simulink library "ePTO"  (R2016a)
settings: Solver=ode45  StartTime=0.0  StopTime=10.0  RelTol=1e-3
undefined symbols (not defined in the file): AWR_InvStError, drvEmot_AWR_InvStError, ePTO, ePTO_baseLoad_enable, ePTO_baseLoad_lutData_power, ePTO_baseLoad_lutIdx_tamb, ePTO_coolingBox_coolingPowerOn, ePTO_coolingBox_coolingPowerStandby, ePTO_coolingBox_enable, ePTO_coolingBox_height, ePTO_coolingBox_isRigid, ePTO_coolingBox_length, ePTO_coolingBox_lowerTemp, ePTO_coolingBox_tempInit, ePTO_coolingBox_tires_rdynTrailer, ePTO_coolingBox_upperTemp, ePTO_coolingBox_width, ePTO_posBasedActivatedConsumer_enable, ePTO_posBasedActivatedConsumer_types, ePTO_triggerBasedActivatedConsumer_enable, ePTO_triggerBasedActivatedConsumer_types
libraries: simulink x5
settings Model: Creator=ORNOVNU  LastModifiedBy=HJAGADI
settings DataIOCC: LimitDataPoints=on  SaveFormat=StructureWithTime
settings HardwareCC: ProdWordSize=32  ProdHWDeviceType=Specified

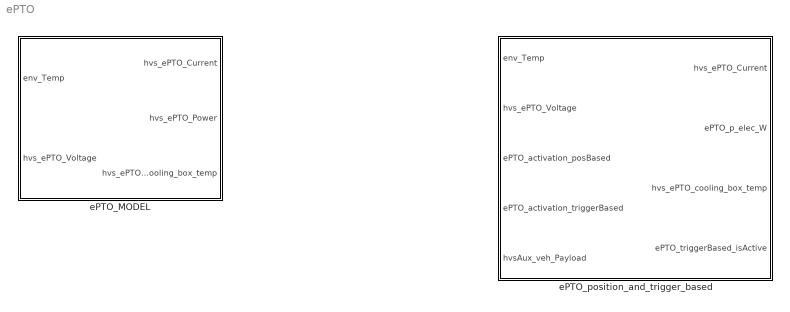
== system ePTO ==
  ePTO_MODEL : Subsystem
  ePTO_position_and_trigger_based : Subsystem

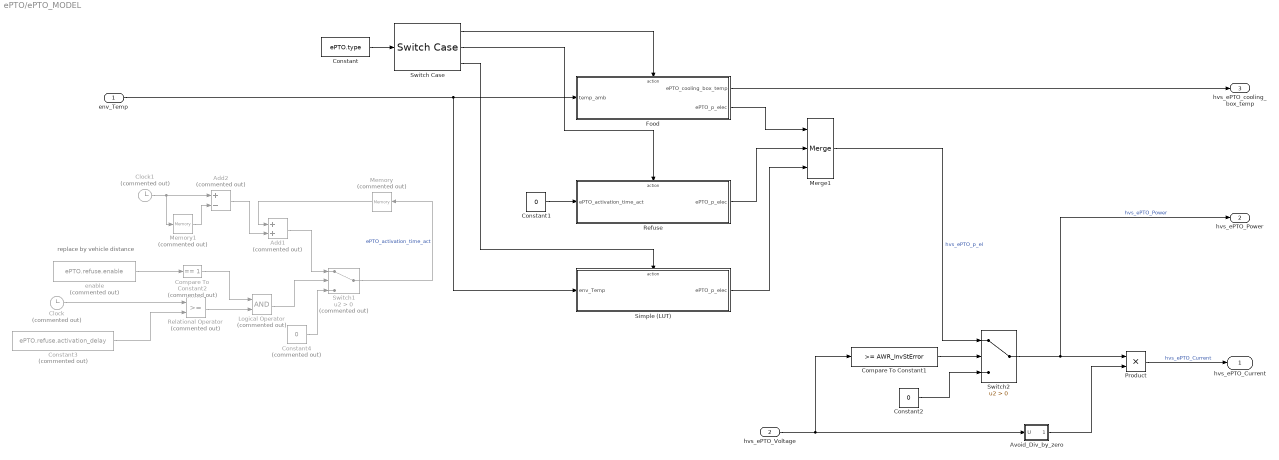
== system ePTO/ePTO_MODEL ==
  note: replace by vehicle distance
  env_Temp : Inport
  hvs_ePTO_Voltage : Inport  Port=2
  Add1 : Sum  Commented=on
  Add2 : Sum  Commented=on  Inputs=+-
  Avoid_Div_by_zero : Subsystem
  Clock : Clock  Commented=on
  Clock1 : Clock  Commented=on
  Compare To Constant1 : simulink/Logic and Bit Operations/Compare To Constant  relop=>=  const=AWR_InvStError  OutDataTypeStr=boolean
  Compare To Constant2 : simulink/Logic and Bit Operations/Compare To Constant  Commented=on  relop===  const=1  OutDataTypeStr=boolean
  Constant : Constant  Value=ePTO.type
  Constant1 : Constant  Value=0
  Constant2 : Constant  Value=0
  Constant3 : Constant  Commented=on  Value=ePTO.refuse.activation_delay
  Constant4 : Constant  Commented=on  Value=0
  Food : Subsystem  TreatAsAtomicUnit=on
  Logical Operator : Logic  Commented=on  AllPortsSameDT=off  OutDataTypeStr=boolean
  Memory : Memory  Commented=on
  Memory1 : Memory  Commented=on
  Merge1 : Merge  Inputs=3
  Product : Product
  Refuse : Subsystem  TreatAsAtomicUnit=on
  Relational Operator : RelationalOperator  Commented=on  OutDataTypeStr=boolean
  Simple (LUT) : Subsystem  TreatAsAtomicUnit=on
  Switch Case : SwitchCase  CaseConditions={1,2}
  Switch1 : Switch  Commented=on  Criteria=u2 > Threshold
  Switch2 : Switch  Criteria=u2 > Threshold
  enable : Constant  Commented=on  Value=ePTO.refuse.enable
  hvs_ePTO_Current : Outport
  hvs_ePTO_Power : Outport  Port=2
  hvs_ePTO_cooling_box_temp : Outport  Port=3
  wires:
  Constant/1 -> Switch Case/1
  Switch Case/1 -> Food/Action
  Switch Case/2 -> Refuse/Action
  Refuse/1(ePTO_p_elec) -> Merge1/2
  Switch1/1 -> Memory/1  "ePTO_activation_time_act"
  enable/1 -> Compare To Constant2/1
  Clock/1 -> Relational Operator/1
  Constant3/1 -> Relational Operator/2
  Constant4/1 -> Switch1/3
  Logical Operator/1 -> Switch1/2
  Relational Operator/1 -> Logical Operator/2
  Compare To Constant2/1 -> Logical Operator/1
  Add2/1 -> Add1/2
  Clock1/1 -> Memory1/1, Add2/1
  Memory1/1 -> Add2/2
  Add1/1 -> Switch1/1
  Memory/1 -> Add1/1
  Constant1/1 -> Refuse/1(ePTO_activation_time_act)
  env_Temp/1 -> Simple (LUT)/1(env_Temp), Food/1(temp_amb)
  Food/2(ePTO_p_elec) -> Merge1/1
  Merge1/1 -> Switch2/1  "hvs_ePTO_p_el"
  Product/1 -> hvs_ePTO_Current/1  "hvs_ePTO_Current"
  Compare To Constant1/1 -> Switch2/2
  Constant2/1 -> Switch2/3
  Food/1(ePTO_cooling_box_temp) -> hvs_ePTO_cooling_box_temp/1
  Switch2/1 -> hvs_ePTO_Power/1, Product/1  "hvs_ePTO_Power"
  hvs_ePTO_Voltage/1 -> Avoid_Div_by_zero/1(U), Compare To Constant1/1
  Avoid_Div_by_zero/1(1/U) -> Product/2
  Switch Case/3 -> Simple (LUT)/Action
  Simple (LUT)/1(ePTO_p_elec) -> Merge1/3

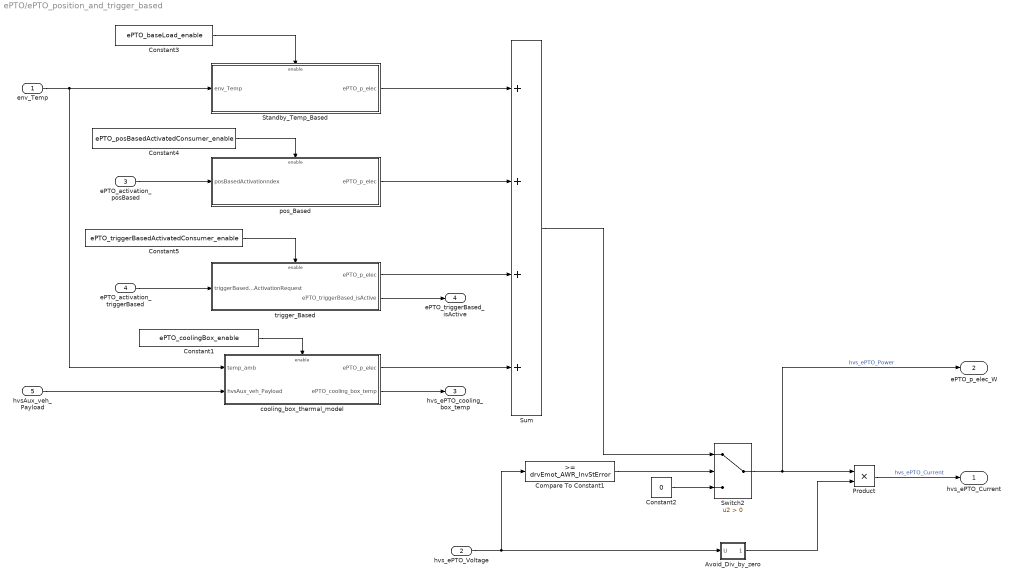
== system ePTO/ePTO_position_and_trigger_based ==
  env_Temp : Inport
  hvs_ePTO_Voltage : Inport  Port=2
  ePTO_activation_posBased : Inport  Port=3
  ePTO_activation_triggerBased : Inport  Port=4
  hvsAux_veh_Payload : Inport  Port=5
  Avoid_Div_by_zero : Subsystem
  Compare To Constant1 : simulink/Logic and Bit Operations/Compare To Constant  relop=>=  const=drvEmot_AWR_InvStError  OutDataTypeStr=boolean
  Constant1 : Constant  Value=ePTO_coolingBox_enable
  Constant2 : Constant  Value=0
  Constant3 : Constant  Value=ePTO_baseLoad_enable
  Constant4 : Constant  Value=ePTO_posBasedActivatedConsumer_enable
  Constant5 : Constant  Value=ePTO_triggerBasedActivatedConsumer_enable
  Product : Product
  Standby_Temp_Based : Subsystem
  Sum : Sum  Inputs=++++
  Switch2 : Switch  Criteria=u2 > Threshold
  cooling_box_thermal_model : Subsystem
  pos_Based : Subsystem
  trigger_Based : Subsystem
  hvs_ePTO_Current : Outport
  ePTO_p_elec_W : Outport  Port=2
  hvs_ePTO_cooling_box_temp : Outport  Port=3
  ePTO_triggerBased_isActive : Outport  Port=4
  wires:
  Avoid_Div_by_zero/1(1/U) -> Product/2
  hvs_ePTO_Voltage/1 -> Avoid_Div_by_zero/1(U), Compare To Constant1/1
  Switch2/1 -> ePTO_p_elec_W/1, Product/1  "hvs_ePTO_Power"
  Constant2/1 -> Switch2/3
  Compare To Constant1/1 -> Switch2/2
  Product/1 -> hvs_ePTO_Current/1  "hvs_ePTO_Current"
  ePTO_activation_posBased/1 -> pos_Based/1(posBasedActivationndex)
  ePTO_activation_triggerBased/1 -> trigger_Based/1(triggerBasedActivationRequest)
  Standby_Temp_Based/1(ePTO_p_elec) -> Sum/1
  trigger_Based/1(ePTO_p_elec) -> Sum/3
  pos_Based/1(ePTO_p_elec) -> Sum/2
  Sum/1 -> Switch2/1
  trigger_Based/2(ePTO_triggerBased_isActive) -> ePTO_triggerBased_isActive/1
  env_Temp/1 -> cooling_box_thermal_model/1(temp_amb), Standby_Temp_Based/1(env_Temp)
  Constant3/1 -> Standby_Temp_Based/Enable
  Constant4/1 -> pos_Based/Enable
  Constant5/1 -> trigger_Based/Enable
  hvsAux_veh_Payload/1 -> cooling_box_thermal_model/2(hvsAux_veh_Payload)
  cooling_box_thermal_model/1(ePTO_p_elec) -> Sum/4
  cooling_box_thermal_model/2(ePTO_cooling_box_temp) -> hvs_ePTO_cooling_box_temp/1
  Constant1/1 -> cooling_box_thermal_model/Enable

== system ePTO/ePTO_MODEL/Avoid_Div_by_zero ==
  U : Inport
  Constant : Constant  Value=10^-6
  Divide : Product  Inputs=/*
  Math Function : Math  Operator=square  SaturateOnIntegerOverflow=on
  Sum : Sum  Inputs=++|
  1/U : Outport
  wires:
  Divide/1 -> 1/U/1
  Math Function/1 -> Divide/1
  Sum/1 -> Divide/2, Math Function/1
  Constant/1 -> Sum/1
  U/1 -> Sum/2

== system ePTO/ePTO_MODEL/Food ==
  temp_amb : Inport
  Action Port : ActionPort  ActionType=case
  ePTO.cooling_box.power_init : Memory
  ePTO.cooling_box.temp_init : Memory  X0=ePTO.cooling_box.temp_init
  ePTO_FOOD_POWER_CALC : Subsystem
  resolve_merge_issue : Gain
  ePTO_cooling_box_temp : Outport
  ePTO_p_elec : Outport  Port=2
  wires:
  ePTO_FOOD_POWER_CALC/1(cooling_box_temp_act) -> ePTO.cooling_box.temp_init/1, ePTO_cooling_box_temp/1
  ePTO.cooling_box.temp_init/1 -> ePTO_FOOD_POWER_CALC/2(cooling_box_temp_act_old)
  ePTO_FOOD_POWER_CALC/2(cooling_box_cooling_power_act) -> resolve_merge_issue/1, ePTO.cooling_box.power_init/1
  ePTO.cooling_box.power_init/1 -> ePTO_FOOD_POWER_CALC/3(cooling_box_cooling_power_act_old)
  temp_amb/1 -> ePTO_FOOD_POWER_CALC/1(env_temp)
  resolve_merge_issue/1 -> ePTO_p_elec/1

== system ePTO/ePTO_MODEL/Refuse ==
  ePTO_activation_time_act : Inport
  Action Port : ActionPort  ActionType=case
  ePTO_rotopress_electric_power : Lookup_n-D  NumberOfTableDimensions=1  BreakpointsForDimension1=ePTO.garbage.time  Table=ePTO.garbage.electric_power  ExtrapMethod=Clip  UseLastTableValue=on  RndMeth=Simplest  InputSameDT=on
  ePTO_p_elec : Outport
  wires:
  ePTO_activation_time_act/1 -> ePTO_rotopress_electric_power/1
  ePTO_rotopress_electric_power/1 -> ePTO_p_elec/1

== system ePTO/ePTO_MODEL/Simple (LUT) ==
  env_Temp : Inport
  Action Port : ActionPort  ActionType=default
  1-D Lookup Table : Lookup_n-D  NumberOfTableDimensions=1  BreakpointsForDimension1=ePTO.simple.lutIdx_tamb  Table=ePTO.simple.lutData_power  ExtrapMethod=Clip  InternalRulePriority=Speed  RndMeth=Simplest  InputSameDT=on
  ePTO_p_elec : Outport
  wires:
  1-D Lookup Table/1 -> ePTO_p_elec/1
  env_Temp/1 -> 1-D Lookup Table/1

== system ePTO/ePTO_position_and_trigger_based/Avoid_Div_by_zero ==
  U : Inport
  Constant : Constant  Value=10^-6
  Divide : Product  Inputs=/*
  Math Function : Math  Operator=square  SaturateOnIntegerOverflow=on
  Sum : Sum  Inputs=++|
  1/U : Outport
  wires:
  U/1 -> Sum/2
  Constant/1 -> Sum/1
  Sum/1 -> Math Function/1, Divide/2
  Math Function/1 -> Divide/1
  Divide/1 -> 1/U/1

== system ePTO/ePTO_position_and_trigger_based/Standby_Temp_Based ==
  env_Temp : Inport
  Enable : EnablePort
  1-D Lookup Table : Lookup_n-D  NumberOfTableDimensions=1  BreakpointsForDimension1=ePTO_baseLoad_lutIdx_tamb  Table=ePTO_baseLoad_lutData_power  ExtrapMethod=Clip  InternalRulePriority=Speed  RndMeth=Simplest  InputSameDT=on
  ePTO_p_elec : Outport
  wires:
  env_Temp/1 -> 1-D Lookup Table/1
  1-D Lookup Table/1 -> ePTO_p_elec/1

== system ePTO/ePTO_position_and_trigger_based/cooling_box_thermal_model ==
  temp_amb : Inport
  hvsAux_veh_Payload : Inport  Port=2
  Enable : EnablePort
  ePTO_FOOD_POWER_CALC : Subsystem
  ePTO_coolingBox_powerInit : Memory  InheritSampleTime=on
  ePTO_coolingBox_tempInit : Memory  X0=ePTO_coolingBox_tempInit  InheritSampleTime=on
  resolve_merge_issue : Gain
  ePTO_p_elec : Outport
  ePTO_cooling_box_temp : Outport  Port=2
  wires:
  ePTO_FOOD_POWER_CALC/1(cooling_box_temp_act) -> ePTO_cooling_box_temp/1, ePTO_coolingBox_tempInit/1
  hvsAux_veh_Payload/1 -> ePTO_FOOD_POWER_CALC/4(hvsAux_veh_Payload)
  resolve_merge_issue/1 -> ePTO_p_elec/1
  ePTO_coolingBox_tempInit/1 -> ePTO_FOOD_POWER_CALC/2(cooling_box_temp_act_old)
  ePTO_FOOD_POWER_CALC/2(cooling_box_cooling_power_act) -> resolve_merge_issue/1, ePTO_coolingBox_powerInit/1
  ePTO_coolingBox_powerInit/1 -> ePTO_FOOD_POWER_CALC/3(cooling_box_cooling_power_act_old)
  temp_amb/1 -> ePTO_FOOD_POWER_CALC/1(env_temp)

== system ePTO/ePTO_position_and_trigger_based/pos_Based ==
  posBasedActivationndex : Inport
  Enable : EnablePort
  Bias : Bias  Bias=-1
  Constant : Constant  Value=0
  Direct Lookup Table (n-D) : LookupNDDirect  NumberOfTableDimensions=1  Table=ePTO_posBasedActivatedConsumer_types
  Saturation1 : Saturate  UpperLimit=99  LowerLimit=1
  Switch : Switch  Criteria=u2 > Threshold
  ePTO_p_elec : Outport
  wires:
  posBasedActivationndex/1 -> Switch/2, Saturation1/1
  Constant/1 -> Switch/3
  Direct Lookup Table (n-D)/1 -> Switch/1
  Switch/1 -> ePTO_p_elec/1
  Bias/1 -> Direct Lookup Table (n-D)/1
  Saturation1/1 -> Bias/1

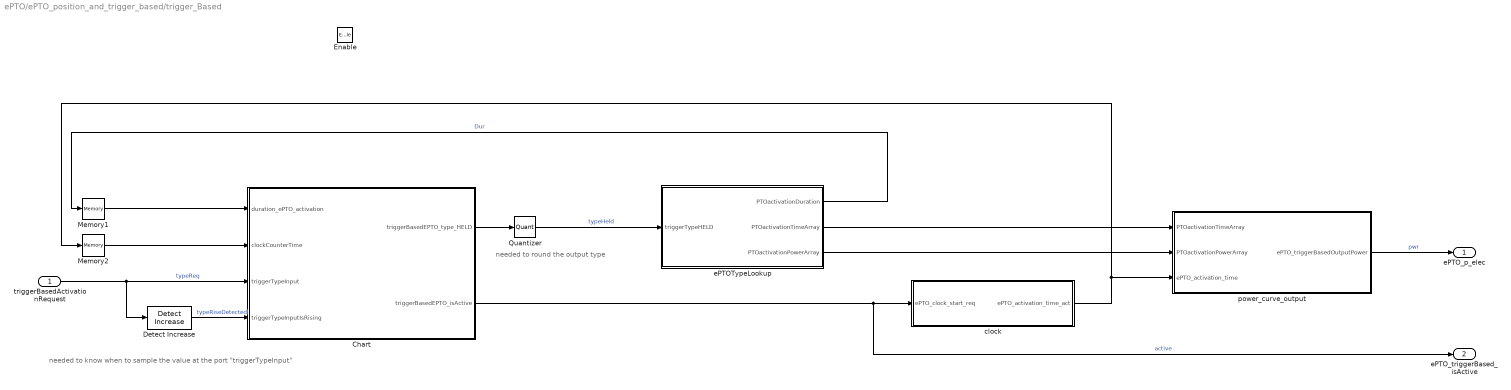
== system ePTO/ePTO_position_and_trigger_based/trigger_Based ==
  note: needed to round the output type
  note: needed to know when to sample the value at the port "triggerTypeInput"
  triggerBasedActivationRequest : Inport
  Enable : EnablePort
  Chart : Stateflow chart  TreatAsAtomicUnit=on
  Detect Increase : simulink/Logic and Bit Operations/Detect Increase  vinit=0.0  OutDataTypeStr=boolean
  Memory1 : Memory  InheritSampleTime=on
  Memory2 : Memory  InheritSampleTime=on
  Quantizer : Quantizer  QuantizationInterval=1
  clock : Subsystem
  ePTOTypeLookup : Subsystem
  power_curve_output : Subsystem
  ePTO_p_elec : Outport
  ePTO_triggerBased_isActive : Outport  Port=2
  wires:
  Memory2/1 -> Chart/2(clockCounterTime)
  clock/1(ePTO_activation_time_act) -> Memory2/1, power_curve_output/3(ePTO_activation_time)
  power_curve_output/1(ePTO_triggerBasedOutputPower) -> ePTO_p_elec/1  "pwr"
  triggerBasedActivationRequest/1 -> Detect Increase/1, Chart/3(triggerTypeInput)  "typeReq"
  ePTOTypeLookup/1(PTOactivationDuration) -> Memory1/1  "Dur"
  ePTOTypeLookup/2(PTOactivationTimeArray) -> power_curve_output/1(PTOactivationTimeArray)
  ePTOTypeLookup/3(PTOactivationPowerArray) -> power_curve_output/2(PTOactivationPowerArray)
  Chart/2(triggerBasedEPTO_isActive) -> ePTO_triggerBased_isActive/1, clock/1(ePTO_clock_start_req)  "active"
  Memory1/1 -> Chart/1(duration_ePTO_activation)
  Chart/1(triggerBasedEPTO_type_HELD) -> Quantizer/1
  Detect Increase/1 -> Chart/4(triggerTypeInputIsRising)  "typeRiseDetected"
  Quantizer/1 -> ePTOTypeLookup/1(triggerTypeHELD)  "typeHeld"

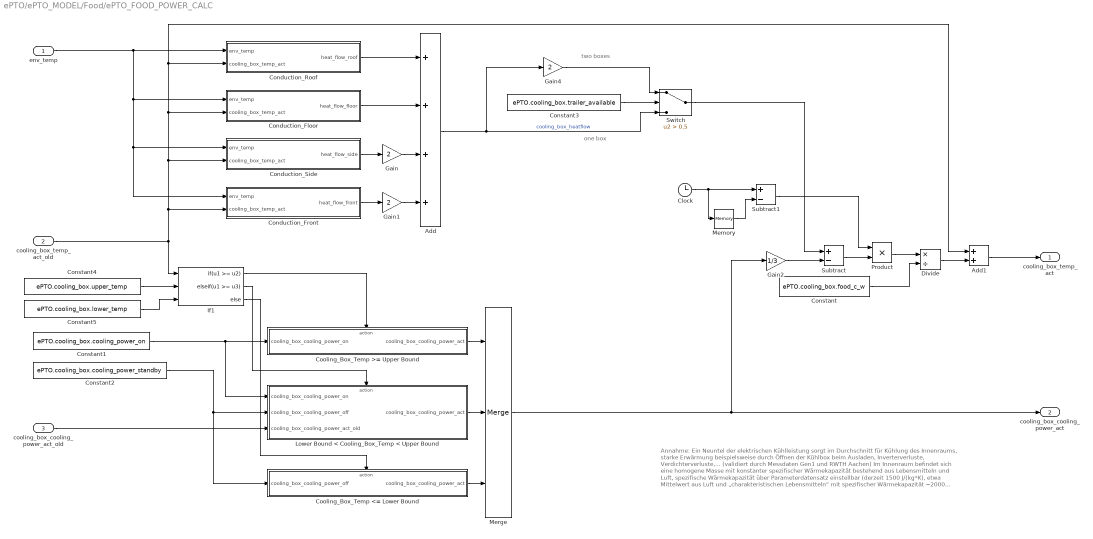
== system ePTO/ePTO_MODEL/Food/ePTO_FOOD_POWER_CALC ==
  note: Annahme: Ein Neuntel der elektrischen Kühlleistung sorgt im Durchschnitt für Kühlung des Innenraums,
      | starke Erwärmung beispielsweise durch Öffnen der Kühlbox beim Ausladen, Inverterverluste, Verdichterverluste,…
      | (validiert durch Messdaten Gen1 und RWTH Aachen)
      |
      | Im Innenraum befindet sich eine homogene Masse mit konstanter spezifischer Wärmekapazität bestehend aus Lebensmitteln und Luft,
      | spezifische Wärmekapazität über Parameterdatensatz einstellbar (derzeit 1500 J/(kg*K),
      | etwa Mittelwert aus Luft und „charakteristischen Lebensmitteln“ mit spezifischer Wärmekapazität ~2000 J/(kg*K)
      |
      | Ref: F. Schuh (TP/EVX)
  note: two boxes
  note: one box
  env_temp : Inport
  cooling_box_temp_act_old : Inport  Port=2
  cooling_box_cooling_power_act_old : Inport  Port=3
  Add : Sum  Inputs=++++
  Add1 : Sum
  Clock : Clock
  Conduction_Floor : Subsystem
  Conduction_Front : Subsystem
  Conduction_Roof : Subsystem
  Conduction_Side : Subsystem
  Constant : Constant  Value=ePTO.cooling_box.food_c_w
  Constant1 : Constant  Value=ePTO.cooling_box.cooling_power_on
  Constant2 : Constant  Value=ePTO.cooling_box.cooling_power_standby
  Constant3 : Constant  Value=ePTO.cooling_box.trailer_available
  Constant4 : Constant  Value=ePTO.cooling_box.upper_temp
  Constant5 : Constant  Value=ePTO.cooling_box.lower_temp
  Cooling_Box_Temp <= Lower Bound : Subsystem  TreatAsAtomicUnit=on
  Cooling_Box_Temp >= Upper Bound : Subsystem  TreatAsAtomicUnit=on
  Divide : Product  Inputs=*/
  Gain : Gain  Gain=2
  Gain1 : Gain  Gain=2
  Gain2 : Gain  Gain=1/3
  Gain4 : Gain  Gain=2
  If1 : If  NumInputs=3  IfExpression=u1 >= u2  ElseIfExpressions=u1 >= u3
  Lower Bound < Cooling_Box_Temp < Upper Bound : Subsystem  TreatAsAtomicUnit=on
  Memory : Memory
  Merge : Merge  Inputs=3
  Product : Product
  Subtract : Sum  Inputs=+-
  Subtract1 : Sum  Inputs=+-
  Switch : Switch  Criteria=u2 > Threshold  Threshold=0.5
  cooling_box_temp_act : Outport
  cooling_box_cooling_power_act : Outport  Port=2
  wires:
  cooling_box_temp_act_old/1 -> If1/1, Conduction_Front/2(cooling_box_temp_act), Conduction_Side/2(cooling_box_temp_act), Conduction_Floor/2(cooling_box_temp_act), Add1/1, Conduction_Roof/2(cooling_box_temp_act)
  Conduction_Side/1(heat_flow_side) -> Gain/1
  Conduction_Front/1(heat_flow_front) -> Gain1/1
  Conduction_Roof/1(heat_flow_roof) -> Add/1
  Conduction_Floor/1(heat_flow_floor) -> Add/2
  Gain/1 -> Add/3
  Gain1/1 -> Add/4
  Add/1 -> Gain4/1, Switch/3  "cooling_box_heatflow"
  Subtract/1 -> Product/2
  Product/1 -> Divide/1
  Constant/1 -> Divide/2
  Divide/1 -> Add1/2
  Add1/1 -> cooling_box_temp_act/1
  If1/1 -> Cooling_Box_Temp >= Upper Bound/Action
  Constant1/1 -> Lower Bound < Cooling_Box_Temp < Upper Bound/1(cooling_box_cooling_power_on), Cooling_Box_Temp >= Upper Bound/1(cooling_box_cooling_power_on)
  If1/2 -> Lower Bound < Cooling_Box_Temp < Upper Bound/Action
  Constant2/1 -> Lower Bound < Cooling_Box_Temp < Upper Bound/2(cooling_box_cooling_power_off), Cooling_Box_Temp <= Lower Bound/1(cooling_box_cooling_power_off)
  If1/3 -> Cooling_Box_Temp <= Lower Bound/Action
  Lower Bound < Cooling_Box_Temp < Upper Bound/1(cooling_box_cooling_power_act) -> Merge/2
  Cooling_Box_Temp >= Upper Bound/1(cooling_box_cooling_power_act) -> Merge/1
  Cooling_Box_Temp <= Lower Bound/1(cooling_box_cooling_power_act) -> Merge/3
  Merge/1 -> cooling_box_cooling_power_act/1, Gain2/1
  Constant3/1 -> Switch/2
  Gain2/1 -> Subtract/2
  env_temp/1 -> Conduction_Floor/1(env_temp), Conduction_Front/1(env_temp), Conduction_Side/1(env_temp), Conduction_Roof/1(env_temp)
  Gain4/1 -> Switch/1
  Switch/1 -> Subtract/1
  Clock/1 -> Memory/1, Subtract1/1
  Memory/1 -> Subtract1/2
  Subtract1/1 -> Product/1
  Constant5/1 -> If1/3
  Constant4/1 -> If1/2
  cooling_box_cooling_power_act_old/1 -> Lower Bound < Cooling_Box_Temp < Upper Bound/3(cooling_box_cooling_power_act_old)

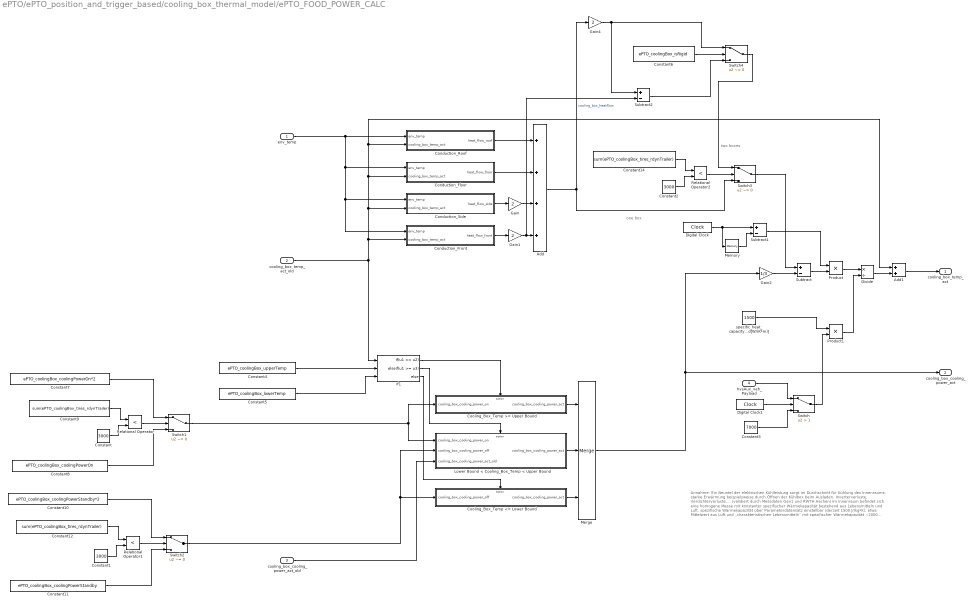
== system ePTO/ePTO_position_and_trigger_based/cooling_box_thermal_model/ePTO_FOOD_POWER_CALC ==
  note: Annahme: Ein Neuntel der elektrischen Kühlleistung sorgt im Durchschnitt für Kühlung des Innenraums,
      | starke Erwärmung beispielsweise durch Öffnen der Kühlbox beim Ausladen, Inverterverluste, Verdichterverluste,…
      | (validiert durch Messdaten Gen1 und RWTH Aachen)
      |
      | Im Innenraum befindet sich eine homogene Masse mit konstanter spezifischer Wärmekapazität bestehend aus Lebensmitteln und Luft,
      | spezifische Wärmekapazität über Parameterdatensatz einstellbar (derzeit 1500 J/(kg*K),
      | etwa Mittelwert aus Luft und „charakteristischen Lebensmitteln“ mit spezifischer Wärmekapazität ~2000 J/(kg*K)
      |
      | Ref: F. Schuh (TP/EVX)
  note: two boxes
  note: one box
  env_temp : Inport
  cooling_box_temp_act_old : Inport  Port=2
  cooling_box_cooling_power_act_old : Inport  Port=3
  hvsAux_veh_Payload : Inport  Port=4
  Add : Sum  Inputs=++++
  Add1 : Sum
  Conduction_Floor : Subsystem
  Conduction_Front : Subsystem
  Conduction_Roof : Subsystem
  Conduction_Side : Subsystem
  Constant : Constant  Value=3000
  Constant1 : Constant  Value=3000
  Constant10 : Constant  Value=ePTO_coolingBox_coolingPowerStandby*2
  Constant11 : Constant  Value=ePTO_coolingBox_coolingPowerStandby
  Constant12 : Constant  Value=sum(ePTO_coolingBox_tires_rdynTrailer)
  Constant14 : Constant  Value=sum(ePTO_coolingBox_tires_rdynTrailer)
  Constant2 : Constant  Value=3000
  Constant3 : Constant  Value=7000
  Constant4 : Constant  Value=ePTO_coolingBox_upperTemp
  Constant5 : Constant  Value=ePTO_coolingBox_lowerTemp
  Constant6 : Constant  Value=ePTO_coolingBox_isRigid
  Constant7 : Constant  Value=ePTO_coolingBox_coolingPowerOn*2
  Constant8 : Constant  Value=ePTO_coolingBox_coolingPowerOn
  Constant9 : Constant  Value=sum(ePTO_coolingBox_tires_rdynTrailer)
  Cooling_Box_Temp <= Lower Bound : Subsystem  TreatAsAtomicUnit=on
  Cooling_Box_Temp >= Upper Bound : Subsystem  TreatAsAtomicUnit=on
  Digital Clock : DigitalClock  SampleTime=-1
  Digital Clock1 : DigitalClock  SampleTime=-1
  Divide : Product  Inputs=*/
  Gain : Gain  Gain=2
  Gain1 : Gain  Gain=2
  Gain2 : Gain  Gain=1/3
  Gain4 : Gain  Gain=2
  If1 : If  NumInputs=3  IfExpression=u1 >= u2  ElseIfExpressions=u1 >= u3
  Lower Bound < Cooling_Box_Temp < Upper Bound : Subsystem  TreatAsAtomicUnit=on
  Memory : Memory  InheritSampleTime=on
  Merge : Merge  Inputs=3
  Product : Product
  Product1 : Product
  Relational Operator : RelationalOperator  Operator=<  OutDataTypeStr=boolean
  Relational Operator1 : RelationalOperator  Operator=<  OutDataTypeStr=boolean
  Relational Operator2 : RelationalOperator  Operator=<  OutDataTypeStr=boolean
  Subtract : Sum  Inputs=+-
  Subtract1 : Sum  Inputs=+-
  Subtract2 : Sum  Inputs=+-
  Switch : Switch  Criteria=u2 > Threshold  Threshold=1
  Switch{1..4} (4 alike) : Switch  Criteria=u2 ~= 0
  specific_heat_capacity_food[W/(K*m)] : Constant  Value=1500
  cooling_box_temp_act : Outport
  cooling_box_cooling_power_act : Outport  Port=2
  wires:
  cooling_box_temp_act_old/1 -> If1/1, Conduction_Front/2(cooling_box_temp_act), Conduction_Side/2(cooling_box_temp_act), Conduction_Floor/2(cooling_box_temp_act), Add1/1, Conduction_Roof/2(cooling_box_temp_act)
  Conduction_Side/1(heat_flow_side) -> Gain/1
  Conduction_Front/1(heat_flow_front) -> Gain1/1
  Conduction_Roof/1(heat_flow_roof) -> Add/1
  Conduction_Floor/1(heat_flow_floor) -> Add/2
  Gain/1 -> Add/3
  Gain1/1 -> Subtract2/2, Add/4
  Add/1 -> Switch3/3, Gain4/1  "cooling_box_heatflow"
  Subtract/1 -> Product/2
  Product/1 -> Divide/1
  Product1/1 -> Divide/2
  Divide/1 -> Add1/2
  Add1/1 -> cooling_box_temp_act/1
  If1/1 -> Cooling_Box_Temp >= Upper Bound/Action
  Switch1/1 -> Lower Bound < Cooling_Box_Temp < Upper Bound/1(cooling_box_cooling_power_on), Cooling_Box_Temp >= Upper Bound/1(cooling_box_cooling_power_on)
  If1/2 -> Lower Bound < Cooling_Box_Temp < Upper Bound/Action
  Switch2/1 -> Lower Bound < Cooling_Box_Temp < Upper Bound/2(cooling_box_cooling_power_off), Cooling_Box_Temp <= Lower Bound/1(cooling_box_cooling_power_off)
  If1/3 -> Cooling_Box_Temp <= Lower Bound/Action
  Lower Bound < Cooling_Box_Temp < Upper Bound/1(cooling_box_cooling_power_act) -> Merge/2
  Cooling_Box_Temp >= Upper Bound/1(cooling_box_cooling_power_act) -> Merge/1
  Cooling_Box_Temp <= Lower Bound/1(cooling_box_cooling_power_act) -> Merge/3
  Merge/1 -> cooling_box_cooling_power_act/1, Gain2/1
  Gain2/1 -> Subtract/2
  env_temp/1 -> Conduction_Floor/1(env_temp), Conduction_Front/1(env_temp), Conduction_Side/1(env_temp), Conduction_Roof/1(env_temp)
  Switch3/1 -> Subtract/1
  Digital Clock/1 -> Memory/1, Subtract1/1
  Memory/1 -> Subtract1/2
  Subtract1/1 -> Product/1
  Constant5/1 -> If1/3
  Constant4/1 -> If1/2
  cooling_box_cooling_power_act_old/1 -> Lower Bound < Cooling_Box_Temp < Upper Bound/3(cooling_box_cooling_power_act_old)
  specific_heat_capacity_food[W/(K*m)]/1 -> Product1/1
  Relational Operator/1 -> Switch1/2
  Constant/1 -> Relational Operator/2
  Constant7/1 -> Switch1/1
  Constant8/1 -> Switch1/3
  Constant9/1 -> Relational Operator/1
  Relational Operator1/1 -> Switch2/2
  Constant1/1 -> Relational Operator1/2
  Constant10/1 -> Switch2/1
  Constant11/1 -> Switch2/3
  Constant12/1 -> Relational Operator1/1
  Relational Operator2/1 -> Switch3/2
  Constant2/1 -> Relational Operator2/2
  Constant14/1 -> Relational Operator2/1
  Digital Clock1/1 -> Switch/2
  hvsAux_veh_Payload/1 -> Switch/1
  Constant3/1 -> Switch/3
  Switch/1 -> Product1/2
  Gain4/1 -> Subtract2/1, Switch4/1
  Switch4/1 -> Switch3/1
  Constant6/1 -> Switch4/2
  Subtract2/1 -> Switch4/3

== system ePTO/ePTO_position_and_trigger_based/trigger_Based/clock ==
  ePTO_clock_start_req : Inport
  Add1 : Sum
  Add2 : Sum  Inputs=+-
  Constant4 : Constant  Value=0
  Digital Clock : DigitalClock  SampleTime=-1
  Memory : Memory  InheritSampleTime=on
  Memory1 : Memory  InheritSampleTime=on
  Switch1 : Switch  Criteria=u2 > Threshold
  ePTO_activation_time_act : Outport
  wires:
  Add1/1 -> Switch1/1
  Memory1/1 -> Add2/2
  Memory/1 -> Add1/1
  Constant4/1 -> Switch1/3
  Switch1/1 -> ePTO_activation_time_act/1, Memory/1  "ePTO_activation_time_act"
  Add2/1 -> Add1/2
  ePTO_clock_start_req/1 -> Switch1/2
  Digital Clock/1 -> Memory1/1, Add2/1

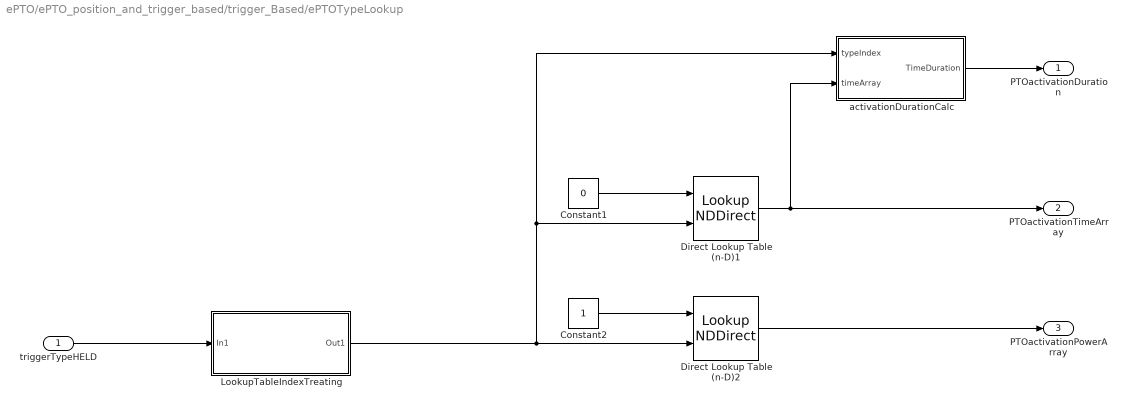
== system ePTO/ePTO_position_and_trigger_based/trigger_Based/ePTOTypeLookup ==
  triggerTypeHELD : Inport
  Constant1 : Constant  Value=0
  Constant2 : Constant
  Direct Lookup Table (n-D)1 : LookupNDDirect  NumberOfTableDimensions=3  InputsSelectThisObjectFromTable=Column  Table=ePTO_triggerBasedActivatedConsumer_types
  Direct Lookup Table (n-D)2 : LookupNDDirect  NumberOfTableDimensions=3  InputsSelectThisObjectFromTable=Column  Table=ePTO_triggerBasedActivatedConsumer_types
  LookupTableIndexTreating : Subsystem
  activationDurationCalc : Subsystem
  PTOactivationDuration : Outport
  PTOactivationTimeArray : Outport  Port=2
  PTOactivationPowerArray : Outport  Port=3
  wires:
  Constant1/1 -> Direct Lookup Table (n-D)1/1
  Constant2/1 -> Direct Lookup Table (n-D)2/1
  Direct Lookup Table (n-D)1/1 -> activationDurationCalc/2(timeArray), PTOactivationTimeArray/1
  Direct Lookup Table (n-D)2/1 -> PTOactivationPowerArray/1
  LookupTableIndexTreating/1(Out1) -> activationDurationCalc/1(typeIndex), Direct Lookup Table (n-D)1/2, Direct Lookup Table (n-D)2/2
  triggerTypeHELD/1 -> LookupTableIndexTreating/1(In1)
  activationDurationCalc/1(TimeDuration) -> PTOactivationDuration/1

== system ePTO/ePTO_position_and_trigger_based/trigger_Based/power_curve_output ==
  PTOactivationTimeArray : Inport
  PTOactivationPowerArray : Inport  Port=2
  ePTO_activation_time : Inport  Port=3
  Lookup Table Dynamic : simulink/Lookup Tables/Lookup Table Dynamic  LookUpMeth=Interpolation-Use End Values  OutDataTypeStr=fixdt('double')  OutputDataTypeScalingMode=Specify via dialog  OutDataType=fixdt('double')  OutScaling=2^-10  DoSatur=off
  ePTO_triggerBasedOutputPower : Outport
  wires:
  ePTO_activation_time/1 -> Lookup Table Dynamic/1
  Lookup Table Dynamic/1 -> ePTO_triggerBasedOutputPower/1
  PTOactivationTimeArray/1 -> Lookup Table Dynamic/2
  PTOactivationPowerArray/1 -> Lookup Table Dynamic/3

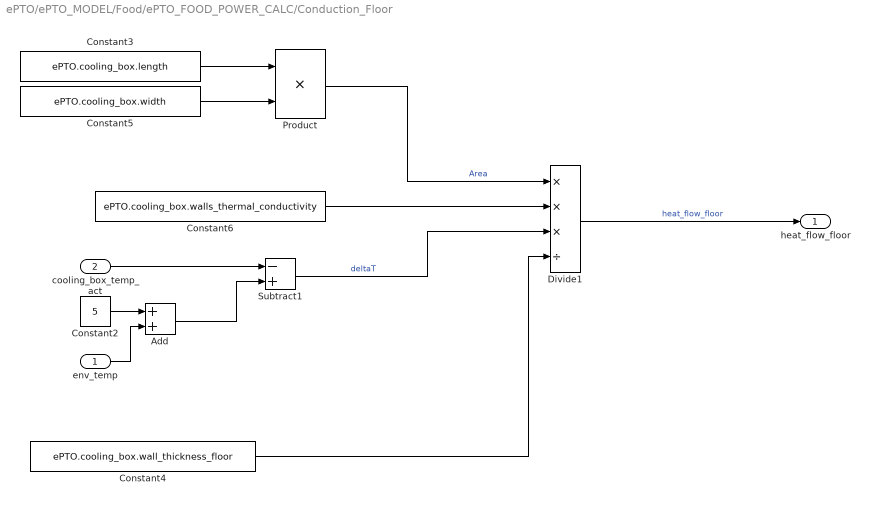
== system ePTO/ePTO_MODEL/Food/ePTO_FOOD_POWER_CALC/Conduction_Floor ==
  env_temp : Inport
  cooling_box_temp_act : Inport  Port=2
  Add : Sum
  Constant2 : Constant  Value=5
  Constant3 : Constant  Value=ePTO.cooling_box.length
  Constant4 : Constant  Value=ePTO.cooling_box.wall_thickness_floor
  Constant5 : Constant  Value=ePTO.cooling_box.width
  Constant6 : Constant  Value=ePTO.cooling_box.walls_thermal_conductivity
  Divide1 : Product  Inputs=***/
  Product : Product
  Subtract1 : Sum  Inputs=-+
  heat_flow_floor : Outport
  wires:
  Divide1/1 -> heat_flow_floor/1  "heat_flow_floor"
  env_temp/1 -> Add/2
  Constant2/1 -> Add/1
  Subtract1/1 -> Divide1/3  "deltaT"
  cooling_box_temp_act/1 -> Subtract1/1
  Product/1 -> Divide1/1  "Area"
  Constant5/1 -> Product/2
  Constant4/1 -> Divide1/4
  Constant3/1 -> Product/1
  Constant6/1 -> Divide1/2
  Add/1 -> Subtract1/2

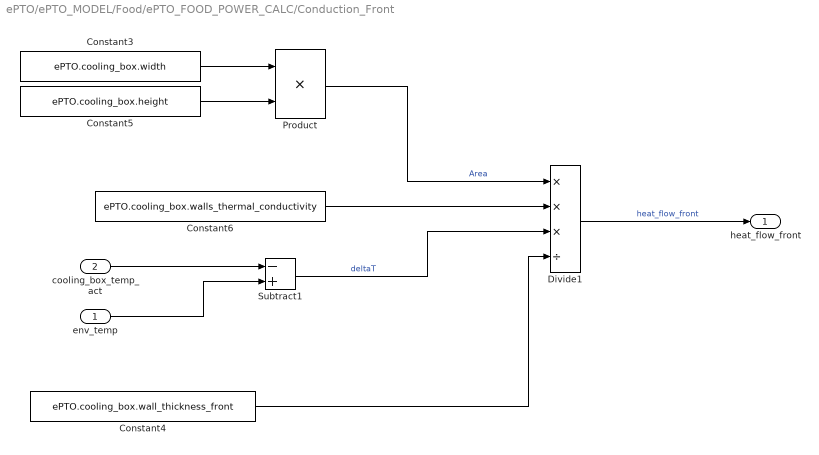
== system ePTO/ePTO_MODEL/Food/ePTO_FOOD_POWER_CALC/Conduction_Front ==
  env_temp : Inport
  cooling_box_temp_act : Inport  Port=2
  Constant3 : Constant  Value=ePTO.cooling_box.width
  Constant4 : Constant  Value=ePTO.cooling_box.wall_thickness_front
  Constant5 : Constant  Value=ePTO.cooling_box.height
  Constant6 : Constant  Value=ePTO.cooling_box.walls_thermal_conductivity
  Divide1 : Product  Inputs=***/
  Product : Product
  Subtract1 : Sum  Inputs=-+
  heat_flow_front : Outport
  wires:
  env_temp/1 -> Subtract1/2
  Product/1 -> Divide1/1  "Area"
  cooling_box_temp_act/1 -> Subtract1/1
  Constant3/1 -> Product/1
  Constant4/1 -> Divide1/4
  Constant6/1 -> Divide1/2
  Subtract1/1 -> Divide1/3  "deltaT"
  Constant5/1 -> Product/2
  Divide1/1 -> heat_flow_front/1  "heat_flow_front"

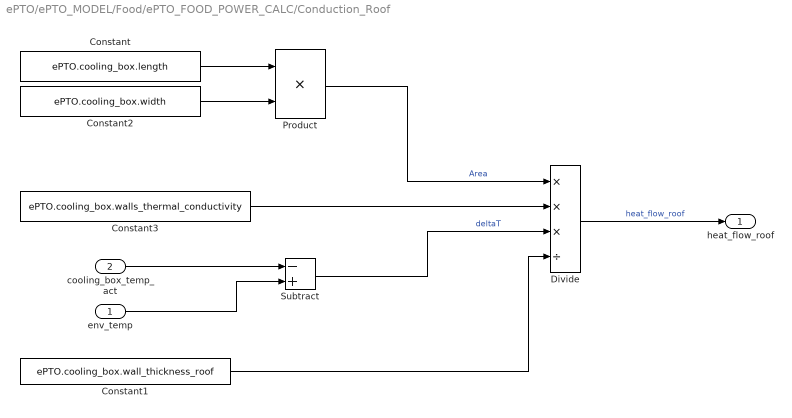
== system ePTO/ePTO_MODEL/Food/ePTO_FOOD_POWER_CALC/Conduction_Roof ==
  env_temp : Inport
  cooling_box_temp_act : Inport  Port=2
  Constant : Constant  Value=ePTO.cooling_box.length
  Constant1 : Constant  Value=ePTO.cooling_box.wall_thickness_roof
  Constant2 : Constant  Value=ePTO.cooling_box.width
  Constant3 : Constant  Value=ePTO.cooling_box.walls_thermal_conductivity
  Divide : Product  Inputs=***/
  Product : Product
  Subtract : Sum  Inputs=-+
  heat_flow_roof : Outport
  wires:
  cooling_box_temp_act/1 -> Subtract/1
  env_temp/1 -> Subtract/2
  Subtract/1 -> Divide/3  "deltaT"
  Divide/1 -> heat_flow_roof/1  "heat_flow_roof"
  Constant/1 -> Product/1
  Constant2/1 -> Product/2
  Product/1 -> Divide/1  "Area"
  Constant1/1 -> Divide/4
  Constant3/1 -> Divide/2

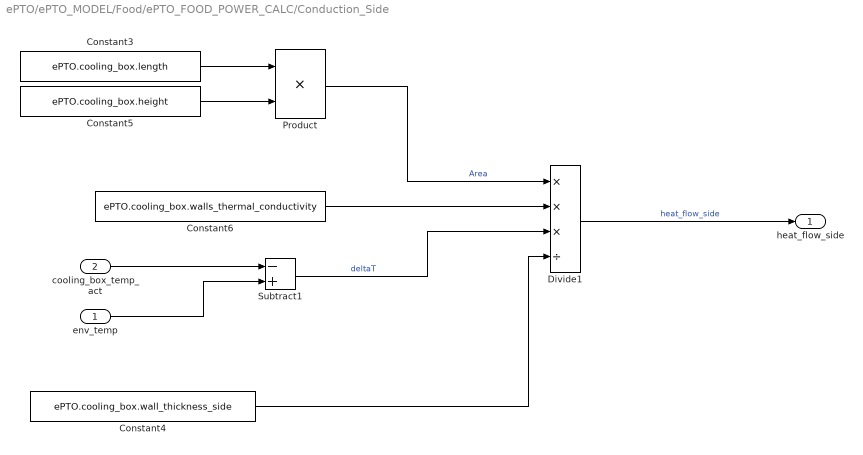
== system ePTO/ePTO_MODEL/Food/ePTO_FOOD_POWER_CALC/Conduction_Side ==
  env_temp : Inport
  cooling_box_temp_act : Inport  Port=2
  Constant3 : Constant  Value=ePTO.cooling_box.length
  Constant4 : Constant  Value=ePTO.cooling_box.wall_thickness_side
  Constant5 : Constant  Value=ePTO.cooling_box.height
  Constant6 : Constant  Value=ePTO.cooling_box.walls_thermal_conductivity
  Divide1 : Product  Inputs=***/
  Product : Product
  Subtract1 : Sum  Inputs=-+
  heat_flow_side : Outport
  wires:
  Constant6/1 -> Divide1/2
  Constant5/1 -> Product/2
  Constant3/1 -> Product/1
  cooling_box_temp_act/1 -> Subtract1/1
  env_temp/1 -> Subtract1/2
  Product/1 -> Divide1/1  "Area"
  Subtract1/1 -> Divide1/3  "deltaT"
  Constant4/1 -> Divide1/4
  Divide1/1 -> heat_flow_side/1  "heat_flow_side"

== system ePTO/ePTO_MODEL/Food/ePTO_FOOD_POWER_CALC/Cooling_Box_Temp <= Lower Bound ==
  cooling_box_cooling_power_off : Inport
  Action Port : ActionPort
  cooling_box_cooling_power_act : Outport
  wires:
  cooling_box_cooling_power_off/1 -> cooling_box_cooling_power_act/1

== system ePTO/ePTO_MODEL/Food/ePTO_FOOD_POWER_CALC/Cooling_Box_Temp >= Upper Bound ==
  cooling_box_cooling_power_on : Inport
  Action Port : ActionPort
  cooling_box_cooling_power_act : Outport
  wires:
  cooling_box_cooling_power_on/1 -> cooling_box_cooling_power_act/1

== system ePTO/ePTO_MODEL/Food/ePTO_FOOD_POWER_CALC/Lower Bound < Cooling_Box_Temp < Upper Bound ==
  cooling_box_cooling_power_on : Inport
  cooling_box_cooling_power_off : Inport  Port=2
  cooling_box_cooling_power_act_old : Inport  Port=3
  Action Port : ActionPort
  Switch : Switch  Criteria=u2 > Threshold  Threshold=ePTO.cooling_box.cooling_power_standby
  cooling_box_cooling_power_act : Outport
  wires:
  cooling_box_cooling_power_on/1 -> Switch/1
  cooling_box_cooling_power_act_old/1 -> Switch/2
  cooling_box_cooling_power_off/1 -> Switch/3
  Switch/1 -> cooling_box_cooling_power_act/1

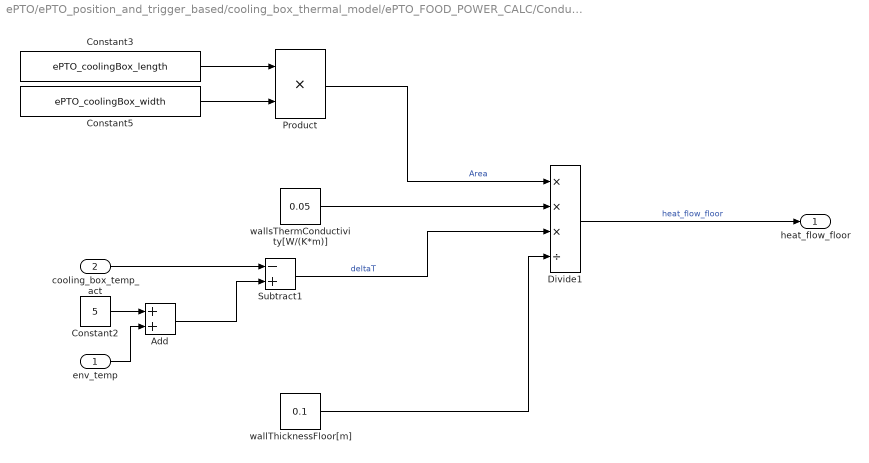
== system ePTO/ePTO_position_and_trigger_based/cooling_box_thermal_model/ePTO_FOOD_POWER_CALC/Conduction_Floor ==
  env_temp : Inport
  cooling_box_temp_act : Inport  Port=2
  Add : Sum
  Constant2 : Constant  Value=5
  Constant3 : Constant  Value=ePTO_coolingBox_length
  Constant5 : Constant  Value=ePTO_coolingBox_width
  Divide1 : Product  Inputs=***/
  Product : Product
  Subtract1 : Sum  Inputs=-+
  "wallThicknessFloor[m] " : Constant  Value=0.1
  wallsThermConductivity[W/(K*m)] : Constant  Value=0.05
  heat_flow_floor : Outport
  wires:
  Divide1/1 -> heat_flow_floor/1  "heat_flow_floor"
  env_temp/1 -> Add/2
  Constant2/1 -> Add/1
  Subtract1/1 -> Divide1/3  "deltaT"
  cooling_box_temp_act/1 -> Subtract1/1
  Product/1 -> Divide1/1  "Area"
  Constant5/1 -> Product/2
  "wallThicknessFloor[m] "/1 -> Divide1/4
  Constant3/1 -> Product/1
  wallsThermConductivity[W/(K*m)]/1 -> Divide1/2
  Add/1 -> Subtract1/2

== system ePTO/ePTO_position_and_trigger_based/cooling_box_thermal_model/ePTO_FOOD_POWER_CALC/Conduction_Front ==
  env_temp : Inport
  cooling_box_temp_act : Inport  Port=2
  Constant3 : Constant  Value=ePTO_coolingBox_width
  Constant5 : Constant  Value=ePTO_coolingBox_height
  Divide1 : Product  Inputs=***/
  Product : Product
  Subtract1 : Sum  Inputs=-+
  wallThicknessFront[m] : Constant  Value=0.055
  wallsThermConductivity[W/(K*m)] : Constant  Value=0.05
  heat_flow_front : Outport
  wires:
  env_temp/1 -> Subtract1/2
  Product/1 -> Divide1/1  "Area"
  cooling_box_temp_act/1 -> Subtract1/1
  Constant3/1 -> Product/1
  wallThicknessFront[m]/1 -> Divide1/4
  wallsThermConductivity[W/(K*m)]/1 -> Divide1/2
  Subtract1/1 -> Divide1/3  "deltaT"
  Constant5/1 -> Product/2
  Divide1/1 -> heat_flow_front/1  "heat_flow_front"

== system ePTO/ePTO_position_and_trigger_based/cooling_box_thermal_model/ePTO_FOOD_POWER_CALC/Conduction_Roof ==
  env_temp : Inport
  cooling_box_temp_act : Inport  Port=2
  Constant : Constant  Value=ePTO_coolingBox_length
  Constant2 : Constant  Value=ePTO_coolingBox_width
  Divide : Product  Inputs=***/
  Product : Product
  Subtract : Sum  Inputs=-+
  wallThicknessRoof[m] : Constant  Value=0.1
  wallsThermConductivity[W/(K*m)] : Constant  Value=0.05
  heat_flow_roof : Outport
  wires:
  cooling_box_temp_act/1 -> Subtract/1
  env_temp/1 -> Subtract/2
  Subtract/1 -> Divide/3  "deltaT"
  Divide/1 -> heat_flow_roof/1  "heat_flow_roof"
  Constant/1 -> Product/1
  Constant2/1 -> Product/2
  Product/1 -> Divide/1  "Area"
  wallThicknessRoof[m]/1 -> Divide/4
  wallsThermConductivity[W/(K*m)]/1 -> Divide/2

== system ePTO/ePTO_position_and_trigger_based/cooling_box_thermal_model/ePTO_FOOD_POWER_CALC/Conduction_Side ==
  env_temp : Inport
  cooling_box_temp_act : Inport  Port=2
  Constant3 : Constant  Value=ePTO_coolingBox_length
  Constant5 : Constant  Value=ePTO_coolingBox_height
  Divide1 : Product  Inputs=***/
  Product : Product
  Subtract1 : Sum  Inputs=-+
  "wallThicknessSide[m] " : Constant  Value=0.055
  wallsThermConductivity[W/(K*m)] : Constant  Value=0.05
  heat_flow_side : Outport
  wires:
  wallsThermConductivity[W/(K*m)]/1 -> Divide1/2
  Constant5/1 -> Product/2
  Constant3/1 -> Product/1
  cooling_box_temp_act/1 -> Subtract1/1
  env_temp/1 -> Subtract1/2
  Product/1 -> Divide1/1  "Area"
  Subtract1/1 -> Divide1/3  "deltaT"
  "wallThicknessSide[m] "/1 -> Divide1/4
  Divide1/1 -> heat_flow_side/1  "heat_flow_side"

== system ePTO/ePTO_position_and_trigger_based/cooling_box_thermal_model/ePTO_FOOD_POWER_CALC/Cooling_Box_Temp <= Lower Bound ==
  cooling_box_cooling_power_off : Inport
  Action Port : ActionPort
  cooling_box_cooling_power_act : Outport
  wires:
  cooling_box_cooling_power_off/1 -> cooling_box_cooling_power_act/1

== system ePTO/ePTO_position_and_trigger_based/cooling_box_thermal_model/ePTO_FOOD_POWER_CALC/Cooling_Box_Temp >= Upper Bound ==
  cooling_box_cooling_power_on : Inport
  Action Port : ActionPort
  cooling_box_cooling_power_act : Outport
  wires:
  cooling_box_cooling_power_on/1 -> cooling_box_cooling_power_act/1

== system ePTO/ePTO_position_and_trigger_based/cooling_box_thermal_model/ePTO_FOOD_POWER_CALC/Lower Bound < Cooling_Box_Temp < Upper Bound ==
  cooling_box_cooling_power_on : Inport
  cooling_box_cooling_power_off : Inport  Port=2
  cooling_box_cooling_power_act_old : Inport  Port=3
  Action Port : ActionPort
  Relational Operator : RelationalOperator  Operator=>  OutDataTypeStr=boolean
  Switch : Switch  Criteria=u2 ~= 0  Threshold=ePTO_coolingBox_coolingPowerStandby
  cooling_box_cooling_power_act : Outport
  wires:
  cooling_box_cooling_power_on/1 -> Switch/1
  Switch/1 -> cooling_box_cooling_power_act/1
  cooling_box_cooling_power_act_old/1 -> Relational Operator/1
  cooling_box_cooling_power_off/1 -> Switch/3, Relational Operator/2
  Relational Operator/1 -> Switch/2

== system ePTO/ePTO_position_and_trigger_based/trigger_Based/ePTOTypeLookup/LookupTableIndexTreating ==
  note: this block is needed, because the lookup table starts with "0" not with "1" (type 1 has an index 0)
      |
      | if index is smaller than 0, type 99 (no power consumption for 1 second) is selected
  In1 : Inport
  Bias : Bias  Bias=-1
  Constant : Constant  Value=99
  Saturation1 : Saturate  UpperLimit=99  LowerLimit=0
  Switch : Switch
  Out1 : Outport
  wires:
  Saturation1/1 -> Bias/1
  Constant/1 -> Switch/3
  In1/1 -> Saturation1/1
  Switch/1 -> Out1/1
  Bias/1 -> Switch/2, Switch/1

== system ePTO/ePTO_position_and_trigger_based/trigger_Based/ePTOTypeLookup/activationDurationCalc ==
  note: Block is neeed to set ePTO activation Duration to 0, if ePTO type is 99
  typeIndex : Inport
  timeArray : Inport  Port=2
  Constant : Constant  Value=0
  Constant3 : Constant  Value=99
  MinMax : MinMax  Function=max
  Relational Operator : RelationalOperator  Operator=<  OutDataTypeStr=boolean
  Switch : Switch  Threshold=99
  TimeDuration : Outport
  wires:
  Switch/1 -> TimeDuration/1
  MinMax/1 -> Switch/1
  Constant/1 -> Switch/3
  Constant3/1 -> Relational Operator/2
  Relational Operator/1 -> Switch/2
  timeArray/1 -> MinMax/1
  typeIndex/1 -> Relational Operator/1

== stateflow chart ePTO/ePTO_position_and_trigger_based/trigger_Based/Chart ==
  state consumer_inactive
    en:
    triggerBasedEPTO_isActive = 0;
    triggerBasedEPTO_type_HELD = 0;
  state rising_edge_detected
  state trigger_input_received
    en:
    triggerBasedEPTO_isActive = 0;
    triggerBasedEPTO_type_HELD = triggerTypeOutput;
  state consumer_active
    en:
    triggerBasedEPTO_isActive = 1;
    triggerBasedEPTO_type_HELD = triggerTypeOutput;
  (default) -> consumer_inactive : {ePTO_cycle_CompleteSts = 0; triggerTypeOutput = 0;}
  consumer_inactive -> consumer_inactive [order 2] : [ePTO_cycle_CompleteSts == 1]
      | {ePTO_cycle_CompleteSts = 0;}
  consumer_active -> consumer_inactive : [clockCounterTime >=  duration_ePTO_activation]
      | {ePTO_cycle_CompleteSts = 1;triggerTypeOutput = 0;}
  consumer_inactive -> rising_edge_detected [order 1] : [hasChangedFrom(triggerTypeInput, 0)]
      | {ePTO_cycle_CompleteSts = 0; }
  rising_edge_detected -> trigger_input_received : [triggerTypeInputIsRising == 0]{triggerTypeOutput = triggerTypeInput; }
  trigger_input_received -> consumer_active : [hasChanged(duration_ePTO_activation)]
  data: duration_ePTO_activation input; clockCounterTime input; triggerTypeInput input; ePTO_cycle_CompleteSts local =0; triggerBasedEPTO_type_HELD output; triggerBasedEPTO_isActive output; triggerTypeOutput local =0; triggerTypeInputIsRising input
